simulink model "robot_traj"  (R2016b)
settings: Solver=ode3  StartTime=0.0  StopTime=1000.0  FixedStep=0.2  RelTol=1e-3  EnableMultiTasking=on
undefined symbols (not defined in the file or in its folder): Angular, Linear
libraries: robotlib x4, simulink x3, realtime_pacer_lib x2
settings Model: Creator=esther  LastModifiedBy=esther
settings DataIOCC: SaveFormat=Array
settings OptimizationCC: MaxStackSize=64
settings DebuggingCC: ParameterTunabilityLossMsg=error
settings HardwareCC: ProdBitPerPointer=32  ProdBitPerSizeT=32  ProdBitPerPtrDiffT=32  ProdLargestAtomicFloat=None  ProdIntDivRoundTo=Undefined  ProdEndianess=Unspecified  ProdWordSize=32  ProdHWDeviceType=Generic->Unspecified (assume 32-bit Generic)
settings RTWCC: SystemTargetFile=ert.tlc  HardwareBoard=Robot Operating System (ROS)  TLCOptions="-aInlineSetEventsForThisBaseRateFcn=TLC_FALSE -aSuppressMultiTaskScheduler=TLC_FALSE  -aRateBasedStepFcn=0"  TemplateMakefile=ert_default_tmf  Description=Embedded Coder  GenerateReport=on  RTWVerbose=off  Toolchain=Catkin  IncludeHyperlinkInReport=on  LaunchReport=on  TargetLang=C++  GenerateTraceInfo=on  GenerateTraceReport=on  GenerateTraceReportSl=on  GenerateTraceReportSf=on  GenerateTraceReportEml=on
settings CodeAppCC: ForceParamTrailComments=on  OperatorAnnotations=on  SimulinkDataObjDesc=on  SFDataObjDesc=on  MATLABFcnDesc=on  InsertBlockDesc=on  MATLABSourceComments=on
settings ERTTargetCC: MultiInstanceERTCode=on  CodeInterfacePackaging=C++ class  SupportContinuousTime=on  SupportVariableSizeSignals=on  RootIOFormat=Structure reference

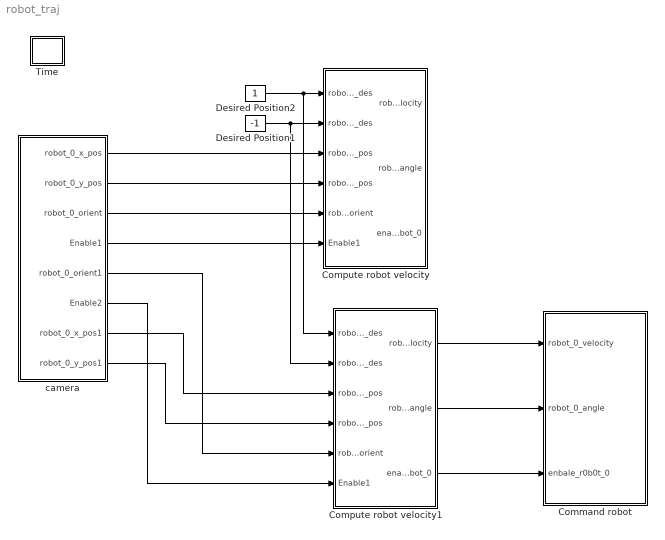
== system robot_traj ==
  Command robot : Subsystem
  Compute robot velocity : Subsystem
  Compute robot velocity1 : Subsystem
  Desired Position1 : Constant  Value=-1  SampleTime=0
  Desired Position2 : Constant  SampleTime=0
  Time : Subsystem
  camera : Subsystem
  wires:
  camera/3(robot_0_orient) -> Compute robot velocity/5(robot_0_orient)
  camera/4(Enable1) -> Compute robot velocity/6(Enable1)
  Desired Position2/1 -> Compute robot velocity1/1(robot_0_x_des), Compute robot velocity/1(robot_0_x_des)
  Desired Position1/1 -> Compute robot velocity/2(robot_0_y_des), Compute robot velocity1/2(robot_0_y_des)
  camera/2(robot_0_y_pos) -> Compute robot velocity/4(robot_0_y_pos)
  camera/1(robot_0_x_pos) -> Compute robot velocity/3(robot_0_x_pos)
  camera/5(robot_0_orient1) -> Compute robot velocity1/5(robot_0_orient)
  camera/6(Enable2) -> Compute robot velocity1/6(Enable1)
  camera/7(robot_0_x_pos1) -> Compute robot velocity1/3(robot_0_x_pos)
  camera/8(robot_0_y_pos1) -> Compute robot velocity1/4(robot_0_y_pos)
  Compute robot velocity1/1(robot_0_velocity) -> Command robot/1(robot_0_velocity)
  Compute robot velocity1/2(robot_0_angle) -> Command robot/2(robot_0_angle)
  Compute robot velocity1/3(enable_robot_0) -> Command robot/3(enbale_r0b0t_0)

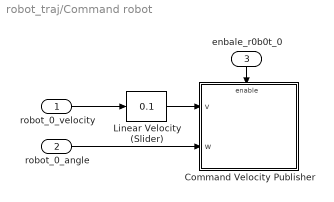
== system robot_traj/Command robot ==
  robot_0_velocity : Inport
  robot_0_angle : Inport  Port=2
  enbale_r0b0t_0 : Inport  Port=3
  Command Velocity Publisher : Subsystem
  Linear Velocity (Slider) : simulink/Math Operations/Slider Gain  low=0  gain=0.1  high=0.2
  wires:
  robot_0_angle/1 -> Command Velocity Publisher/2(w)
  enbale_r0b0t_0/1 -> Command Velocity Publisher/Enable
  robot_0_velocity/1 -> Linear Velocity (Slider)/1
  Linear Velocity (Slider)/1 -> Command Velocity Publisher/1(v)

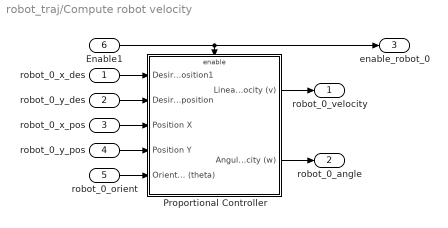
== system robot_traj/Compute robot velocity ==
  robot_0_x_des : Inport
  robot_0_y_des : Inport  Port=2
  robot_0_x_pos : Inport  Port=3
  robot_0_y_pos : Inport  Port=4
  robot_0_orient : Inport  Port=5
  Enable1 : Inport  Port=6
  Proportional Controller : Subsystem
  robot_0_velocity : Outport
  robot_0_angle : Outport  Port=2
  enable_robot_0 : Outport  Port=3
  wires:
  Proportional Controller/1(Linear Velocity (v)) -> robot_0_velocity/1
  Proportional Controller/2(Angular Velocity (w)) -> robot_0_angle/1
  robot_0_x_pos/1 -> Proportional Controller/3(Position X)
  robot_0_orient/1 -> Proportional Controller/5(Orientation (theta))
  robot_0_x_des/1 -> Proportional Controller/1(Desired position1)
  robot_0_y_pos/1 -> Proportional Controller/4(Position Y)
  robot_0_y_des/1 -> Proportional Controller/2(Desired position)
  Enable1/1 -> enable_robot_0/1, Proportional Controller/Enable

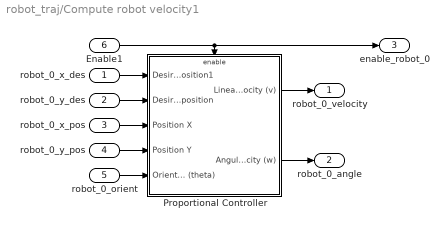
== system robot_traj/Compute robot velocity1 ==
  robot_0_x_des : Inport
  robot_0_y_des : Inport  Port=2
  robot_0_x_pos : Inport  Port=3
  robot_0_y_pos : Inport  Port=4
  robot_0_orient : Inport  Port=5
  Enable1 : Inport  Port=6
  Proportional Controller : Subsystem
  robot_0_velocity : Outport
  robot_0_angle : Outport  Port=2
  enable_robot_0 : Outport  Port=3
  wires:
  Proportional Controller/1(Linear Velocity (v)) -> robot_0_velocity/1
  Proportional Controller/2(Angular Velocity (w)) -> robot_0_angle/1
  robot_0_x_pos/1 -> Proportional Controller/3(Position X)
  robot_0_orient/1 -> Proportional Controller/5(Orientation (theta))
  robot_0_x_des/1 -> Proportional Controller/1(Desired position1)
  robot_0_y_pos/1 -> Proportional Controller/4(Position Y)
  robot_0_y_des/1 -> Proportional Controller/2(Desired position)
  Enable1/1 -> enable_robot_0/1, Proportional Controller/Enable

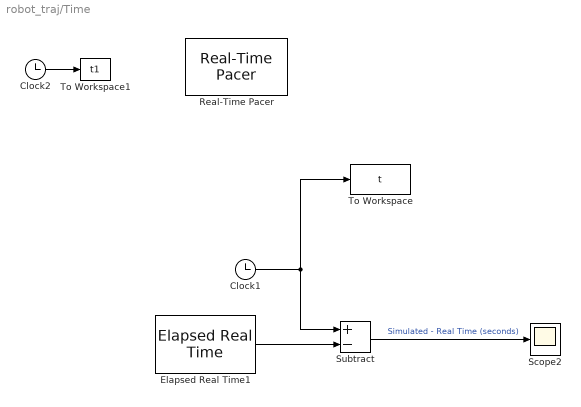
== system robot_traj/Time ==
  Clock1 : Clock
  Clock2 : Clock
  Elapsed Real Time1 : realtime_pacer_lib/Elapsed Real Time
  Real-Time Pacer : realtime_pacer_lib/Real-Time Pacer  simTimePerRealTime=1
  Scope2 : Scope
  Subtract : Sum  Inputs=+-
  To Workspace : ToWorkspace  VariableName=t  SaveFormat=Timeseries  SampleTime=-1
  To Workspace1 : ToWorkspace  VariableName=t1  SampleTime=-1
  wires:
  Elapsed Real Time1/1 -> Subtract/2
  Subtract/1 -> Scope2/1  "Simulated - Real Time (seconds)"
  Clock1/1 -> To Workspace/1, Subtract/1
  Clock2/1 -> To Workspace1/1

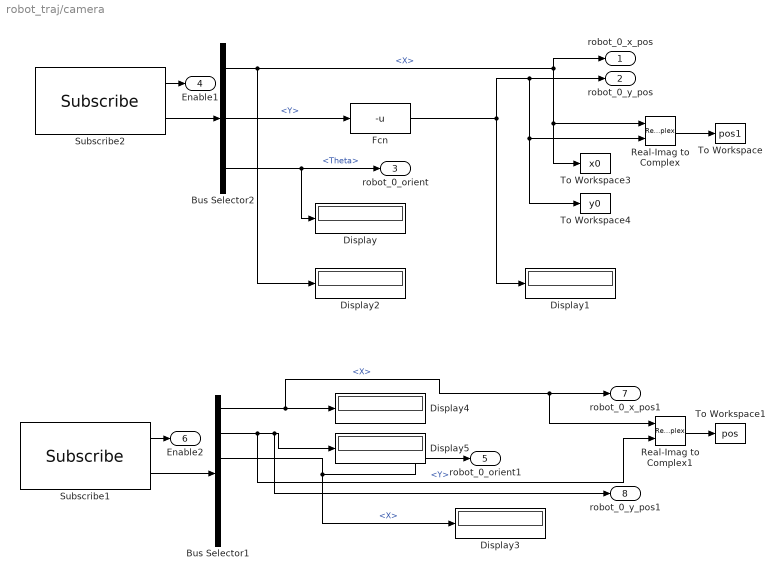
== system robot_traj/camera ==
  Bus Selector1 : BusSelector  OutputSignals=Pose.Pose.Position.X,Pose.Pose.Position.Y,Pose.Pose.Orientation.X,Pose.Pose.Orientation.Y,Pose.Pose.Orientation.Z,Pose.Pose.Orientation.W
  Bus Selector2 : BusSelector  OutputSignals=X,Y,Theta
  Display{,1..5} (6 alike) : Display
  Fcn : Fcn  Expr=-u
  Real-Imag to Complex : RealImagToComplex
  Real-Imag to Complex1 : RealImagToComplex
  Subscribe1 : robotlib/Subscribe  SourceLibraryInfo=This block requires Robotics System Toolbox  topicSource=Select from ROS network  topic=/robot_0/pose  messageType=nav_msgs/Odometry  sampleTime=-1  messageQueueLength=1
  Subscribe2 : robotlib/Subscribe  SourceLibraryInfo=This block requires Robotics System Toolbox  topicSource=Select from ROS network  topic=/bot_0/ground_pose  messageType=geometry_msgs/Pose2D  sampleTime=-1  messageQueueLength=1
  To Workspace : ToWorkspace  VariableName=pos1  SampleTime=-1
  To Workspace1 : ToWorkspace  VariableName=pos  SampleTime=-1
  To Workspace3 : ToWorkspace  VariableName=x0  SampleTime=-1
  To Workspace4 : ToWorkspace  VariableName=y0  SampleTime=-1
  robot_0_x_pos : Outport
  robot_0_y_pos : Outport  Port=2
  robot_0_orient : Outport  Port=3
  Enable1 : Outport  Port=4
  robot_0_orient1 : Outport  Port=5
  Enable2 : Outport  Port=6
  robot_0_x_pos1 : Outport  Port=7
  robot_0_y_pos1 : Outport  Port=8
  wires:
  Subscribe2/2 -> Bus Selector2/1
  Subscribe2/1 -> Enable1/1
  Real-Imag to Complex/1 -> To Workspace/1
  Bus Selector2/1 -> Display2/1, robot_0_x_pos/1, Real-Imag to Complex/1, To Workspace3/1  "<X>"
  Bus Selector2/2 -> Fcn/1  "<Y>"
  Bus Selector2/3 -> robot_0_orient/1, Display/1  "<Theta>"
  ? -> ?  "<Y>"
  Fcn/1 -> robot_0_y_pos/1, Real-Imag to Complex/2, To Workspace4/1, Display1/1
  Subscribe1/2 -> Bus Selector1/1
  Subscribe1/1 -> Enable2/1
  Bus Selector1/1 -> Real-Imag to Complex1/1, robot_0_x_pos1/1, Display4/1  "<X>"
  Bus Selector1/2 -> Real-Imag to Complex1/2, robot_0_y_pos1/1, Display5/1  "<Y>"
  Bus Selector1/3 -> Display3/1, robot_0_orient1/1  "<X>"
  Real-Imag to Complex1/1 -> To Workspace1/1

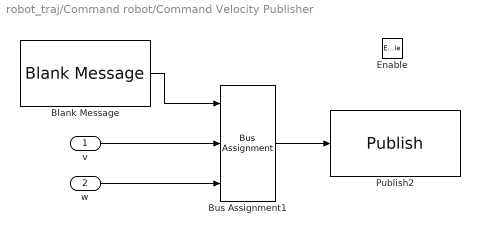
== system robot_traj/Command robot/Command Velocity Publisher ==
  v : Inport
  w : Inport  Port=2
  Enable : EnablePort
  Blank Message : robotlib/Blank Message  SourceLibraryInfo=This block requires Robotics System Toolbox  messageType=geometry_msgs/Twist  SampleTime=inf
  Bus Assignment1 : BusAssignment  DialogController=Simulink.DDGSource_BusAssignment  AssignedSignals=Linear.X,Angular.Z
  Publish2 : robotlib/Publish  SourceLibraryInfo=This block requires Robotics System Toolbox  topicSource=Select from ROS network  topic=/robot_0/cmd_vel  messageType=geometry_msgs/Twist  messageQueueLength=105
  wires:
  Bus Assignment1/1 -> Publish2/1
  Blank Message/1 -> Bus Assignment1/1
  v/1 -> Bus Assignment1/2
  w/1 -> Bus Assignment1/3

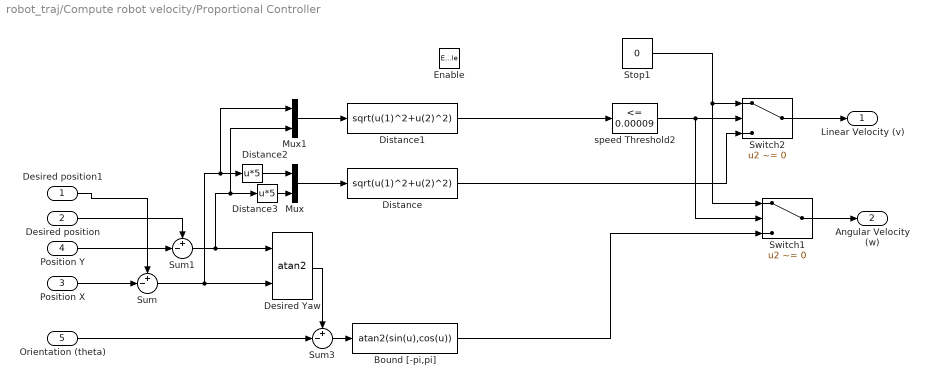
== system robot_traj/Compute robot velocity/Proportional Controller ==
  Desired position1 : Inport
  Desired position : Inport  Port=2
  Position X : Inport  Port=3
  Position Y : Inport  Port=4
  Orientation (theta) : Inport  Port=5
  Enable : EnablePort
  Bound [-pi,pi] : Fcn  Expr=atan2(sin(u),cos(u))
  Desired Yaw : Trigonometry  Operator=atan2
  Distance : Fcn  Expr=sqrt(u(1)^2+u(2)^2)
  Distance1 : Fcn  Expr=sqrt(u(1)^2+u(2)^2)
  Distance2 : Fcn  Expr=u*5
  Distance3 : Fcn  Expr=u*5
  Mux : Mux  Inputs=2
  Mux1 : Mux  Inputs=2
  Stop1 : Constant  Value=0
  Sum : Sum  Inputs=+-|
  Sum1 : Sum  Inputs=+-|
  Sum3 : Sum  Inputs=+-|
  Switch1 : Switch  Criteria=u2 ~= 0
  Switch2 : Switch  Criteria=u2 ~= 0
  speed Threshold2 : simulink/Logic and Bit Operations/Compare To Constant  relop=<=  const=0.00009  OutDataTypeStr=boolean
  Linear Velocity (v) : Outport
  Angular Velocity (w) : Outport  Port=2
  wires:
  Desired position1/1 -> Sum/1
  Desired position/1 -> Sum1/1
  Position Y/1 -> Sum1/2
  Position X/1 -> Sum/2
  Mux/1 -> Distance/1
  Orientation (theta)/1 -> Sum3/2
  Desired Yaw/1 -> Sum3/1
  Sum3/1 -> Bound [-pi,pi]/1
  Distance/1 -> Switch2/3
  Distance2/1 -> Mux/1
  Distance3/1 -> Mux/2
  Mux1/1 -> Distance1/1
  Sum/1 -> Desired Yaw/2, Mux1/1, Distance2/1
  Sum1/1 -> Desired Yaw/1, Mux1/2, Distance3/1
  speed Threshold2/1 -> Switch2/2, Switch1/2
  Bound [-pi,pi]/1 -> Switch1/3
  Stop1/1 -> Switch2/1, Switch1/1
  Distance1/1 -> speed Threshold2/1
  Switch1/1 -> Angular Velocity (w)/1
  Switch2/1 -> Linear Velocity (v)/1

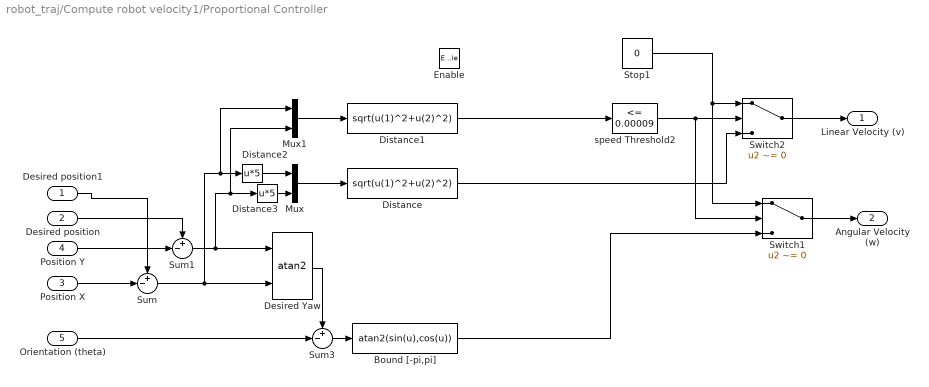
== system robot_traj/Compute robot velocity1/Proportional Controller ==
  Desired position1 : Inport
  Desired position : Inport  Port=2
  Position X : Inport  Port=3
  Position Y : Inport  Port=4
  Orientation (theta) : Inport  Port=5
  Enable : EnablePort
  Bound [-pi,pi] : Fcn  Expr=atan2(sin(u),cos(u))
  Desired Yaw : Trigonometry  Operator=atan2
  Distance : Fcn  Expr=sqrt(u(1)^2+u(2)^2)
  Distance1 : Fcn  Expr=sqrt(u(1)^2+u(2)^2)
  Distance2 : Fcn  Expr=u*5
  Distance3 : Fcn  Expr=u*5
  Mux : Mux  Inputs=2
  Mux1 : Mux  Inputs=2
  Stop1 : Constant  Value=0
  Sum : Sum  Inputs=+-|
  Sum1 : Sum  Inputs=+-|
  Sum3 : Sum  Inputs=+-|
  Switch1 : Switch  Criteria=u2 ~= 0
  Switch2 : Switch  Criteria=u2 ~= 0
  speed Threshold2 : simulink/Logic and Bit Operations/Compare To Constant  relop=<=  const=0.00009  OutDataTypeStr=boolean
  Linear Velocity (v) : Outport
  Angular Velocity (w) : Outport  Port=2
  wires:
  Desired position1/1 -> Sum/1
  Desired position/1 -> Sum1/1
  Position Y/1 -> Sum1/2
  Position X/1 -> Sum/2
  Mux/1 -> Distance/1
  Orientation (theta)/1 -> Sum3/2
  Desired Yaw/1 -> Sum3/1
  Sum3/1 -> Bound [-pi,pi]/1
  Distance/1 -> Switch2/3
  Distance2/1 -> Mux/1
  Distance3/1 -> Mux/2
  Mux1/1 -> Distance1/1
  Sum/1 -> Desired Yaw/2, Mux1/1, Distance2/1
  Sum1/1 -> Desired Yaw/1, Mux1/2, Distance3/1
  speed Threshold2/1 -> Switch2/2, Switch1/2
  Bound [-pi,pi]/1 -> Switch1/3
  Stop1/1 -> Switch2/1, Switch1/1
  Distance1/1 -> speed Threshold2/1
  Switch1/1 -> Angular Velocity (w)/1
  Switch2/1 -> Linear Velocity (v)/1
